simulink model "test_heater_model"  (R2014b)
settings: Solver=ode45  StartTime=0.0  StopTime=40  RelTol=1e-3
values from neighbouring files (symbols this model uses):
  a1 = c(1)    [Model.m]
  a2 = c(2)    [Model.m]
  a3 = d(1)    [Model.m]
  a4 = d(2)    [Model.m]
  d = C\D    [Model.m]
libraries: simulink x1
settings Model: Creator=Admin  LastModifiedBy=Admin

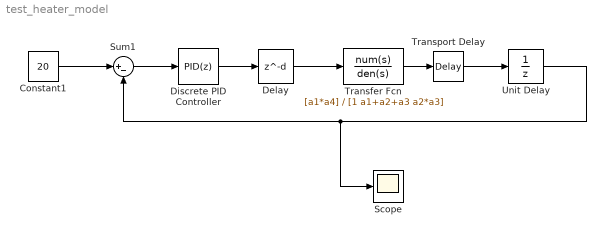
== system test_heater_model ==
  Constant1 : Constant  Value=20
  Delay : Delay  DelayLength=d
  Discrete PID Controller : simulink/Continuous/PID Controller  Controller=PID  TimeDomain=Discrete-time  SampleTime=1  IntegratorMethod=Forward Euler  FilterMethod=Forward Euler  Form=Parallel  P=40.4324549268521  I=2.49124466610014  D=80.8959370764653  N=1.67342543377406  InitialConditionSource=internal  InitialConditionForIntegrator=0  InitialConditionForFilter=0  ExternalReset=none  LimitOutput=off  UpperSaturationLimit=inf  LowerSaturationLimit=-inf  LinearizeAsGain=off  AntiWindupMode=none  Kb=1  TrackingMode=off  Kt=1  PParamMin=[]  PParamMax=[]  IParamMin=[]  IParamMax=[]  DParamMin=[]  DParamMax=[]  NParamMin=[]  NParamMax=[]  KbParamMin=[]  KbParamMax=[]  KtParamMin=[]  KtParamMax=[]  POutMin=[]  POutMax=[]  IOutMin=[]  IOutMax=[]  DOutMin=[]  DOutMax=[]  NOutMin=[]  NOutMax=[]  KbOutMin=[]  KbOutMax=[]  KtOutMin=[]  KtOutMax=[]  IntegratorOutMin=[]  IntegratorOutMax=[]  FilterOutMin=[]  FilterOutMax=[]  SumOutMin=[]  SumOutMax=[]  SumI1OutMin=[]  SumI1OutMax=[]  SumI2OutMin=[]  SumI2OutMax=[]  SumI3OutMin=[]  SumI3OutMax=[]  SumDOutMin=[]  SumDOutMax=[]  SaturationOutMin=[]  SaturationOutMax=[]  IntegratorContinuousStateAttributes=''  IntegratorStateMustResolveToSignalObject=off  IntegratorRTWStateStorageClass=Auto  FilterContinuousStateAttributes=''  FilterStateMustResolveToSignalObject=off  FilterRTWStateStorageClass=Auto  DifferentiatorICPrevScaledInput=0  DifferentiatorOutMin=[]  DifferentiatorOutMax=[]  UseFilter=on
  Scope : Scope
  Sum1 : Sum  Inputs=|+-
  Transfer Fcn : TransferFcn  Numerator=[a1*a4]  Denominator=[1 a1+a2+a3 a2*a3]
  Transport Delay : TransportDelay
  Unit Delay : UnitDelay  SampleTime=-1
  wires:
  Transfer Fcn/1 -> Transport Delay/1
  Transport Delay/1 -> Unit Delay/1
  Delay/1 -> Transfer Fcn/1
  Discrete PID Controller/1 -> Delay/1
  Constant1/1 -> Sum1/1
  Unit Delay/1 -> Scope/1, Sum1/2
  Sum1/1 -> Discrete PID Controller/1
